simulink model "ship_5_kalman_release"  (Simulink 8.6)
settings: Solver=ode45  StartTime=0.0  StopTime=600  RelTol=1e-3
values from neighbouring files (symbols this model uses):
  K_pd = sqrt((omega_c^2 * T_f)^2 + omega_c^2) / K    [boat_3.m]
  T_d = T    (= 86.5246)    [boat_3.m]
  T_f = 1/(omega_c * tan(deg2rad(50)))    [boat_3.m]
libraries: simulink_extras x2, simulink x1
settings Model: Creator=markh  LastModifiedBy=Bernt Johan
settings DataIOCC: SignalLoggingName=sigsOut
settings OptimizationCC: ExpressionDepthLimit=128  InitFltsAndDblsToZero=on
settings DebuggingCC: SaveWithParameterizedLinksMsg=none  SignalResolutionControl=TryResolveAllWithWarning  SolverPrmCheckMsg=none  MultiTaskDSMMsg=warning  MultiTaskCondExecSysMsg=none  FcnCallInpInsideContextMsg=UseLocalSettings
settings HardwareCC: TargetUnknown=on
settings GRTTargetCC: TargetFcnLib=ansi_tfl_tmw.mat

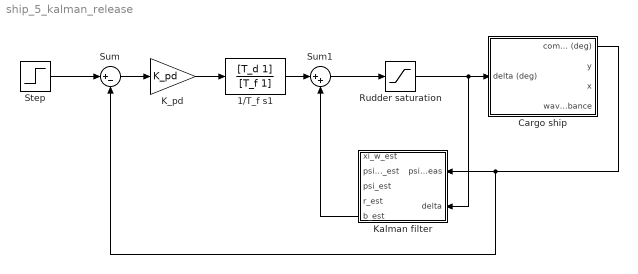
== system ship_5_kalman_release ==
  1/T_f s1 : TransferFcn  Numerator=[T_d 1]  Denominator=[T_f 1]
  Cargo ship : Subsystem  mask(Simple shipmodel for a cargo ship){noise=on, current=on, logic=on}
      mask prompts: noise "measurement noise"; logic "waves"
      mask help:
      | Measurement noise:
      | 	checked = noise on
      | 	unchecked = noise off
      |
      | Current:
      | 	checked = current on
      | 	unchecked = current off
      |
      | Waves:
      | 	checked = waves on
      | 	unchecked = waves off
      |
      | Author: Jørgen Spjøtvold, 9/10-2003
      | TTK 4115 Linear system theory.
      | Modified by Jostein Bakkeheim 26/10-2006
  K_pd : Gain  Gain=K_pd
  Kalman filter : Subsystem
  Rudder saturation : Saturate  UpperLimit=45  LowerLimit=-45
  Step : Step  Time=0  After=30  SampleTime=0
  Sum : Sum  Inputs=|+-
  Sum1 : Sum  Inputs=|++
  wires:
  Step/1 -> Sum/1
  Sum/1 -> K_pd/1
  Rudder saturation/1 -> Kalman filter/2(delta), Cargo ship/1(delta (deg))
  K_pd/1 -> 1/T_f s1/1
  Sum1/1 -> Rudder saturation/1
  1/T_f s1/1 -> Sum1/1
  Kalman filter/5(b_est) -> Sum1/2
  Cargo ship/1(compass (deg)) -> Sum/2, Kalman filter/1(psi_meas)

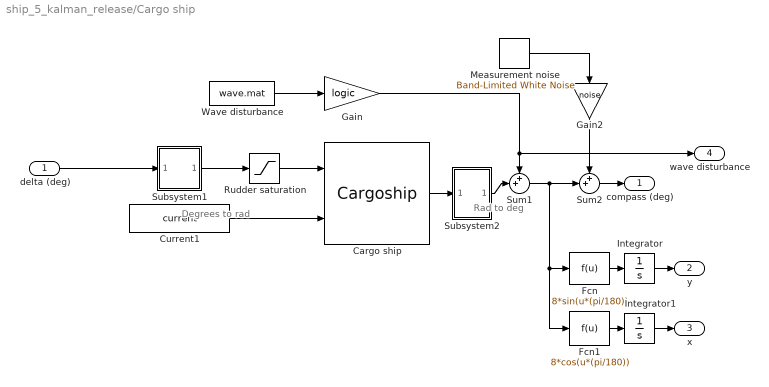
== system ship_5_kalman_release/Cargo ship ==
  note: Degrees to rad
  note: Rad to deg
  delta (deg) : Inport
  Cargo ship : S-Function  FunctionName=Cargoship  SFunctionDeploymentMode=off  EnableBusSupport=off  mask(Cargo ship){}
      mask help:
      | S-function which simulates a cargo ship.
      |
      | Author: Jørgen Spjøtvold
      | 20.10-2003
      | Modified by Jostein Bakkeheim 27.10.2006
  Current1 : Constant  Value=current
  Fcn : Fcn  Expr=8*sin(u*(pi/180))
  Fcn1 : Fcn  Expr=8*cos(u*(pi/180))
  Gain : Gain  Gain=logic  SaturateOnIntegerOverflow=on  OutDataTypeStr=Inherit: Same as input  ParamDataTypeStr=Inherit: Same as input
  Gain2 : Gain  Gain=noise  SaturateOnIntegerOverflow=on  OutDataTypeStr=Inherit: Same as input  ParamDataTypeStr=Inherit: Same as input
  Integrator : Integrator
  Integrator1 : Integrator
  Measurement noise : simulink/Sources/Band-Limited White Noise  Cov=[0.001]  Ts=.5  seed=[23341]
  Rudder saturation : Saturate  UpperLimit=45*(pi/180)  LowerLimit=-45*(pi/180)
  Subsystem1 : Subsystem  mask(degrees to radians){}
      mask help: Converts degrees to radians
      mask Display: fprintf('D2R');
  Subsystem2 : Subsystem  mask(radians to degrees){}
      mask help: Converts radians to degrees
      mask Display: fprintf('R2D');
  Sum1 : Sum  Inputs=++|  SaturateOnIntegerOverflow=on
  Sum2 : Sum  Inputs=++|  SaturateOnIntegerOverflow=on
  Wave disturbance : FromFile  FileName=wave.mat  SampleTime=0
  compass (deg) : Outport
  y : Outport  Port=2
  x : Outport  Port=3
  "wave disturbance " : Outport  Port=4
  wires:
  delta (deg)/1 -> Subsystem1/1(In1)
  Fcn/1 -> Integrator/1
  Integrator/1 -> y/1
  Fcn1/1 -> Integrator1/1
  Integrator1/1 -> x/1
  Wave disturbance/1 -> Gain/1
  Subsystem2/1(Out1) -> Sum1/2
  Gain/1 -> "wave disturbance "/1, Sum1/1
  Sum1/1 -> Fcn/1, Fcn1/1, Sum2/2
  Cargo ship/1 -> Subsystem2/1(In1)
  Subsystem1/1(Out1) -> Rudder saturation/1
  Rudder saturation/1 -> Cargo ship/1
  Sum2/1 -> compass (deg)/1
  Measurement noise/1 -> Gain2/1
  Gain2/1 -> Sum2/1
  Current1/1 -> Cargo ship/2

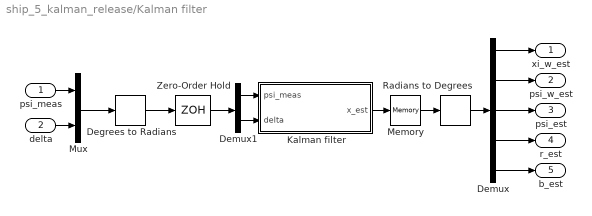
== system ship_5_kalman_release/Kalman filter ==
  psi_meas : Inport
  delta : Inport  Port=2
  Degrees to Radians : simulink_extras/Transformations/Degrees to Radians
  Demux : Demux  Outputs=5
  Demux1 : Demux  Outputs=2
  Kalman filter : MATLAB Function  TreatAsAtomicUnit=on
  Memory : Memory
  Mux : Mux  Inputs=2
  Radians to Degrees : simulink_extras/Transformations/Radians to Degrees
  Zero-Order Hold : ZeroOrderHold  SampleTime=0.1
  xi_w_est : Outport  PortDimensions=1
  psi_w_est : Outport  Port=2  PortDimensions=1
  psi_est : Outport  Port=3  PortDimensions=1
  r_est : Outport  Port=4  PortDimensions=1
  b_est : Outport  Port=5  PortDimensions=1
  wires:
  Mux/1 -> Degrees to Radians/1
  psi_meas/1 -> Mux/1
  delta/1 -> Mux/2
  Radians to Degrees/1 -> Demux/1
  Degrees to Radians/1 -> Zero-Order Hold/1
  Demux1/1 -> Kalman filter/1(psi_meas)
  Demux1/2 -> Kalman filter/2(delta)
  Zero-Order Hold/1 -> Demux1/1
  Kalman filter/1(x_est) -> Memory/1
  Demux/5 -> b_est/1
  Demux/4 -> r_est/1
  Demux/3 -> psi_est/1
  Demux/2 -> psi_w_est/1
  Demux/1 -> xi_w_est/1
  Memory/1 -> Radians to Degrees/1

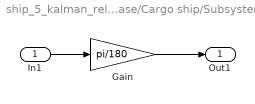
== system ship_5_kalman_release/Cargo ship/Subsystem1 ==
  In1 : Inport
  Gain : Gain  Gain=pi/180  SaturateOnIntegerOverflow=on  OutDataTypeStr=Inherit: Same as input  ParamDataTypeStr=Inherit: Same as input
  Out1 : Outport
  wires:
  Gain/1 -> Out1/1
  In1/1 -> Gain/1

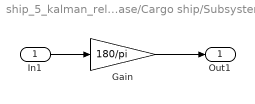
== system ship_5_kalman_release/Cargo ship/Subsystem2 ==
  In1 : Inport
  Gain : Gain  Gain=180/pi  SaturateOnIntegerOverflow=on  OutDataTypeStr=Inherit: Same as input  ParamDataTypeStr=Inherit: Same as input
  Out1 : Outport
  wires:
  Gain/1 -> Out1/1
  In1/1 -> Gain/1

== matlab function Kalman filter/Kalman filter ==
  data: psi_meas input double; x_est output double; delta input double
function x_est  = kalman_m( psi_meas, delta )
%KALMAN_M Kalman filter
%   Detailed explanation goes here
Ad = [0.996954741048002,0.0992545087604663,0,0,0;-0.0607430933636516,0.984111959963574,0,0,0;0,0,1,0.0999422352218680,-1.00626243505991e-05;0,0,0,0.998844926931510,-0.000201213728530954;0,0,0,0,1];
Bd = [0;0;1.006262435059909e-05;2.012137285309542e-04;0];
Cd = [0,1,1,0,0];
Ed = [2.487983938514842e-05,0;4.962725438023313e-04,0;0,-3.354531141537223e-07;0,-1.006262435059910e-05;0,0.100000000000000];
R = 6.092300000000000e-07;
Q = [30 0; 0 1e-6];
persistent x_est_pre P_est_pre init_flag
if isempty(init_flag)
    init_flag = 1;
    x_est_pre = [0;0;0;0;0];
    P_est_pre = diag([1 0.013 pi^2 1 2.5e-4]);
end

K = P_est_pre*transpose(Cd)/(Cd*P_est_pre*transpose(Cd) + R);
x_est = x_est_pre + K * (psi_meas - Cd*x_est_pre);
x_est_pre = Ad*x_est + Bd*delta;
P_est = (eye(5)-K*Cd)*P_est_pre*transpose(eye(5)-K*Cd) + K*R*transpose(K);
P_est_pre = Ad*P_est*transpose(Ad) + Ed*Q*transpose(Ed);
